simulink model "CONTROL_SYSTEM_V3"  (R2024a)
settings: Solver=FixedStepAuto  StartTime=0.0  StopTime=inf  FixedStep=0.01  RelTol=1e-3
values from neighbouring files (symbols this model uses):
  Beta1 = 3*Omega_o    (= 15)    [CONTROL_SYSTEM_VAR.m]
  Beta2 = 3*(Omega_o^2)    (= 75)    [CONTROL_SYSTEM_VAR.m]
  Beta3 = (Omega_o^3)    (= 125)    [CONTROL_SYSTEM_VAR.m]
  Desire_Max = 255    [CONTROL_SYSTEM_VAR.m]
  Desire_Min = 0    [CONTROL_SYSTEM_VAR.m]
  Direction_Pin = 1    [CONTROL_SYSTEM_VAR.m]
  EN_Pin = 0    [CONTROL_SYSTEM_VAR.m]
  J_aet = 0.0035    [CONTROL_SYSTEM_VAR.m]
  Kd = 2    [CONTROL_SYSTEM_VAR.m]
  Ki = 4    [CONTROL_SYSTEM_VAR.m]
  Kn = 0.1    [CONTROL_SYSTEM_VAR.m]
  Kp = 1.4    [CONTROL_SYSTEM_VAR.m]
  omga_c = 10    [CONTROL_SYSTEM_VAR.m]
  roa = 0.24    [CONTROL_SYSTEM_VAR.m]
undefined symbols (not defined in the file or in its folder): sigbuilder_block
libraries: arduinolib x30, simulink_extras x14, simulink x5, slpidlib x4, SignalEditorBlockLib x3, slctrl_adaptive x2, spsOnDelayLib x2, slctrl_autotuning x2
(part 1 of 5)
settings Model: ExtModeTrigDuration=2  Creator=Banana444  LastModifiedBy=Banana444
settings SolverCC: AutoInsertRateTranBlk=on
settings OptimizationCC: EnhancedBackFolding=on  PassReuseOutputArgsAs=Individual arguments  ZeroExternalMemoryAtStartup=off  ZeroInternalMemoryAtStartup=off  MaxStackSize=64  OptimizeBlockOrder=speed  DifferentSizesBufferReuse=on  OptimizationCustomize=off  EfficientTunableParamExpr=on
settings DebuggingCC: ParameterTunabilityLossMsg=error
settings HardwareCC: ProdBitPerPointer=32  ProdBitPerSizeT=32  ProdBitPerPtrDiffT=32  ProdLargestAtomicInteger=Long  ProdLargestAtomicFloat=Double  ProdWordSize=32  ProdHWDeviceType=ARM Compatible->ARM Cortex
settings SFSimCC: MATLABDynamicMemAlloc=off
settings RTWCC: Description=Embedded Coder  SystemTargetFile=ert.tlc  HardwareBoard=ESP32-WROOM(Arduino Compatible)  TLCOptions="-aInlineSetEventsForThisBaseRateFcn=TLC_FALSE -aSuppressMultiTaskScheduler=TLC_FALSE  -aRateBasedStepFcn=0"  TemplateMakefile=ert_default_tmf  Toolchain=ESP32
settings CodeAppCC: ForceParamTrailComments=on  IgnoreCustomStorageClasses=off  OperatorAnnotations=on  SimulinkDataObjDesc=on  SFDataObjDesc=on  InsertBlockDesc=on
settings ERTTargetCC: SupportContinuousTime=on  SupportVariableSizeSignals=on  ExtModeTransport=3  ExtModeStaticAlloc=on  ExtModeAutomaticAllocSize=off  ExtModeStaticAllocSize=65536  ExtModeMexFile=ext_xcp  ExtModeIntrfLevel=Level2 - Open

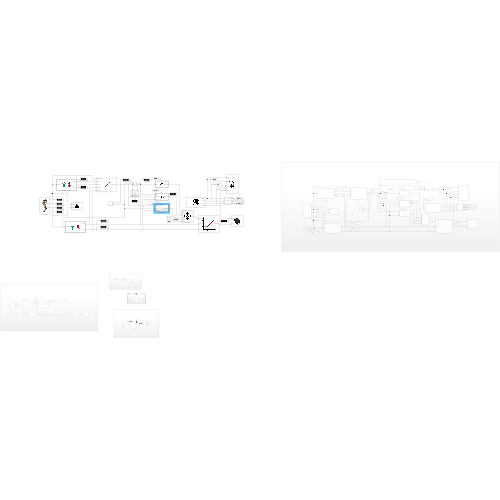
[thumbnail: Simulink's stored preview of the top-level diagram]
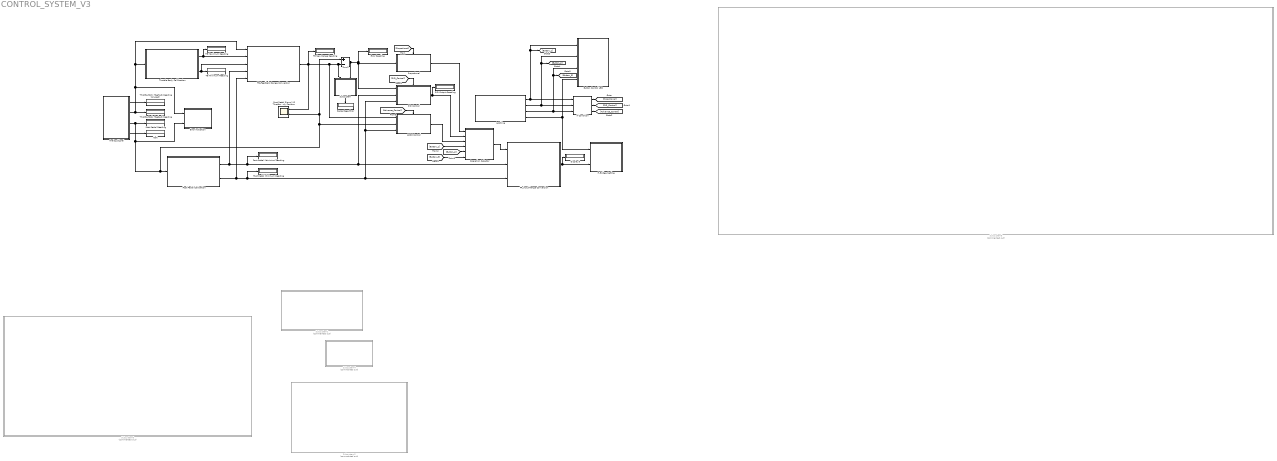
== system CONTROL_SYSTEM_V3 ==
  ADRC Control : Subsystem
  Analog Signal : Subsystem
      mask Display: image('Capture.JPG', [0,0,0,0,80,80]);
  Button Control LED : Subsystem
      mask Display: image('LED.png', [0,0,0,0,80,80]);
  Display3 : Display
      settings: Decimation=2
  Error Indication : Subsystem
      settings: PortSchema="{\"entries\":[{\"content\":{\"sides\":[{\"content\":{},\"type\":\"ConnectorPlacement.EquallySpacedRectSide\",\"uuid\":\"6bb27259-0fc4-412b-bd28-187413250838\"},{\"content\":{\"connectorIds\":[\"In1\",\"In2\"],\"side\":\"RIGHT\"},\"type\":\"ConnectorPlacement.EquallySpacedRectSide\",\"uuid\":\"b38a583a-7cdb-4b72-8a0e-445370b0f03f\"},{\"content\":{\"side\":\"TOP\"},\"type\":\"ConnectorPlacement.EquallySpacedRectSide\",\"uuid\":\"477ad40e-8e68-4653-afaf-50b4ab734c9d\"}]},\"type\":\"ConnectorPlacement.EquallySpacedConnector\",\"uuid\":\"474c0f68-6b48-44ee-b6ec-af4e49acdc40\"}],\"packageUris\":[\"http://schema.mathworks.com/mf0/Connector/R2020b\"],\"version\":\"1.0\"}"
      mask Display: image('Waring.png', [0,0,0,0,80,80]);
  Error Reading : Display
      settings: Decimation=2
  FP_Input Range Conversion : Subsystem
      mask Display: image('Interpolation.png', [0,0,0,0,80,80]);
  Foot Pedal Calibration : MATLAB Function  TreatAsAtomicUnit=on
  Foot Pedal Maximum Reading : Display
      settings: Decimation=2
  Foot Pedal Minimum Reading : Display
      settings: Decimation=2
  Foot Pedal Reading : Display
      settings: Decimation=2
  Foot Pedal Signal VS Throttle Body Position : Scope  NumInputPorts=2
  H-Bridge Setting : Subsystem
      mask Display: image('H-Bridge-removebg-preview.png', [0,0,0,0,80,80]);
  If Condition : If  NumInputs=3  IfExpression=u1 == 1  ElseIfExpressions=u2 == 1, u3 == 1  ShowElse=off
  Latching : Subsystem
      mask Display: image('Switch.png', [0,0,0,0,80,80]);
  NaN : Display
      settings: Decimation=2
  Operation Selector : Subsystem
      mask Display: image('Decision.png', [0,0,0,0,80,80]);
  PID Control : Subsystem
      mask Display: image('PID.PNG', [0,0,0,0,50,50]);
  PID Output Reading : Display
      settings: Decimation=2
  Percentage Error : Display
      settings: Decimation=2
  Propotional : Subsystem  TreatAsAtomicUnit=on
      mask Display: image('Propotional.png', [0,0,0,0,80,80]);
  Subsystem : Subsystem
      settings: PortSchema="{\"entries\":[{\"content\":{\"sides\":[{\"content\":{},\"type\":\"ConnectorPlacement.EquallySpacedRectSide\",\"uuid\":\"06ab9b8c-dc11-4e78-9aea-2a49b899d383\"},{\"content\":{\"side\":\"RIGHT\"},\"type\":\"ConnectorPlacement.EquallySpacedRectSide\",\"uuid\":\"ea81575a-6f3e-44ea-98d6-a15110b05ea2\"},{\"content\":{\"connectorIds\":[\"In1\",\"In2\"],\"side\":\"TOP\"},\"type\":\"ConnectorPlacement.EquallySpacedRectSide\",\"uuid\":\"b4582e74-93d2-4cba-bd7b-a3215d2fef1c\"},{\"content\":{\"connectorIds\":[\"Out1\"],\"side\":\"BOTTOM\"},\"type\":\"ConnectorPlacement.EquallySpacedRectSide\",\"uuid\":\"d3012ec7-4a68-4cee-bd0d-e63c4f089545\"}]},\"type\":\"ConnectorPlacement.EquallySpacedConnector\",\"uuid\":\"85ff3d74-6a46-44e9-8a38-f9999c5d3ee8\"}],\"packageUris\":[\"http://schema.mathworks.com/mf0/Connector/R2020b\"],\"version\":\"1.0\"}"
  Subsystem1 : Subsystem  Commented=on
  Subsystem2 : Subsystem  Commented=on
  Subsystem4 : Subsystem  Commented=on
  Subsystem5 : Subsystem  Commented=on
  Subsystem6 : Subsystem  Commented=on
  Sum2 : Sum  Inputs=+-
  TB Maximum Reading : Display
      settings: Decimation=2
  TB Minimum Reading : Display
      settings: Decimation=2
  TB New Range Reading : Display
      settings: Decimation=2
  TB_Feedbakc Range Conversion : Subsystem
      mask Display: image('Interpolation.png', [0,0,0,0,80,80]);
  Throttle Body Callibration : MATLAB Function  TreatAsAtomicUnit=on
  Throttle Body Feeback Reading : Display
      settings: Decimation=2
  Throttle Body Feeback Reading (Unused) : Display
      settings: Decimation=2
  wires:
  ADRC Control/1(ADRC Output) -> Operation Selector/3(Advanced Control)
  Propotional/1(Propotional) -> Operation Selector/1(Propotional)
  [Button_1] -> Operation Selector/4(Switch 1)
  Subsystem/1(Percentage Error) -> Percentage Error/1  "Percentage Error"
  Latching/3(Button 3) -> If Condition/3, [Button_3], Button Control LED/3(Button 3)
  [Advance_Control] -> ADRC Control/Action
  If Condition/2 -> [PID_Control]
  If Condition/1 -> [Propotional]
  [Propotional] -> Propotional/Action
  [Button_3] -> Operation Selector/6(Switch 3)
  TB_Feedbakc Range Conversion/1(TB New Range) -> Sum2/2, Subsystem/1(Throttle Body Feedback), ADRC Control/1(Feedback), Foot Pedal Signal VS Throttle Body Position/1, TB New Range Reading/1  "Throttle Body Feedback"
  Sum2/1 -> PID Control/1(Error), Propotional/1(Error), Error Reading/1, Subsystem/2(In1)  "Error"
  Throttle Body Callibration/1(TB_maxVal) -> TB Maximum Reading/1, TB_Feedbakc Range Conversion/2(TB_maxVal)
  Operation Selector/1(Control Output) -> FP_Input Range Conversion/1(Control Output)
  PID Control/1(PID Output) -> Operation Selector/2(PID Output), PID Output Reading/1
  Analog Signal/3(PedalRange) -> ADRC Control/2(Desire), Foot Pedal Signal VS Throttle Body Position/2, Sum2/1, Foot Pedal Calibration/1(PedalRange), Error Indication/1(PedalRange), Foot Pedal Reading/1  "Foot Pedal Signal"
  Foot Pedal Calibration/1(FP_maxVal) -> FP_Input Range Conversion/2(FP_maxVal), PID Control/2(FP_maxVal), Foot Pedal Maximum Reading/1, TB_Feedbakc Range Conversion/4(FP_maxVal)
  [Button_2] -> Operation Selector/5(Switch 2)
  If Condition/3 -> [Advance_Control]
  Analog Signal/4(Out4) -> NaN/1
  FP_Input Range Conversion/1(0 - 255 Output) -> H-Bridge Setting/2(0 - 255), Display3/1
  Latching/1(Button 1) -> [Button_1], Button Control LED/1(Button 1), If Condition/1
  Foot Pedal Calibration/2(FP_minVal) -> FP_Input Range Conversion/3(FP_minVal), ADRC Control/3(FP_minVal), PID Control/3(FP_minVal), Foot Pedal Minimum Reading/1, TB_Feedbakc Range Conversion/5(FP_minVal)
  Analog Signal/1(Out1) -> Throttle Body Feeback Reading (Unused)/1
  [PID_Control] -> PID Control/Action
  Latching/4(Button 4) -> H-Bridge Setting/1(Calibration Mode), Button Control LED/4(Button 4)
  Analog Signal/2(TBRange) -> Throttle Body Feeback Reading/1, Error Indication/2(TBRange), Throttle Body Callibration/1(TB_Range), TB_Feedbakc Range Conversion/1(Control Output)
  Throttle Body Callibration/2(TB_minVal) -> TB Minimum Reading/1, TB_Feedbakc Range Conversion/3(TB_minVal)
  Latching/2(Button 2) -> [Button_2], Button Control LED/2(Bottun 2), If Condition/2

== system CONTROL_SYSTEM_V3/ADRC Control ==
  Feedback : Inport
  Desire : Inport  Port=2
  FP_minVal : Inport  Port=3
  Action Port : ActionPort  ActionPortLabel=elseif( u3 == 1)
  Active Disturbance Rejection Control : slctrl_adaptive/Active Disturbance Rejection Control  time_domain=continuous-time  Ts=-1  model_type=second-order  b0=1000  wc=5  wo=5*8  x0=0  ulim_checkbox=off  umax=inf  umin=-inf  xhat_checkbox=off
      settings: LibrarySourceBlock=slctrlblks/Adaptive Control/Active Disturbance Rejection Control
  Constant : Constant  Value=2
  Divide : Product  Inputs=*/
  Saturation Dynamic : simulink/Discontinuities/Saturation Dynamic  OutMin=[]  OutMax=[]  OutDataTypeStr=Inherit: Same as second input  OutDataType=fixdt(1, 16)  OutScaling=2^-10  DoSatur=off
  Subsystem : Subsystem  Commented=on
  Sum1 : Sum  Inputs=++|
  ADRC Output : Outport
  wires:
  FP_minVal/1 -> Saturation Dynamic/3
  Subsystem/1(V(t)) -> ?
  Sum1/1 -> Saturation Dynamic/1
  Constant/1 -> Divide/2
  Active Disturbance Rejection Control/1 -> Saturation Dynamic/2
  Feedback/1 -> Active Disturbance Rejection Control/2
  Desire/1 -> Divide/1, Sum1/2, Active Disturbance Rejection Control/1
  Saturation Dynamic/1 -> ADRC Output/1
  Divide/1 -> Sum1/1

== system CONTROL_SYSTEM_V3/Analog Signal ==
  note: Analog Read Custom Block reaading;
      | - Throttle Body Feedback (V1)
      | - Foot Padel Signal (V2)
  MATLAB System : MATLABSystem  System=ADS1115_Vread  SetGain=int16( 16 )  SampleTime=-1
      mask Type: ADS1115_Vread
      mask Display:
      | color('white');plot([100,100,100,100]*1,[100,100,100,100]*1);plot([100,100,100,100]*0,[100,100,100,100]*0);color('blue');text(38, 92, 'IO Device Builder','horizontalAlignment', 'right');
      | color('black');text(52,50,' ADS1115_Vread','horizontalAlignment','center');
      | port_label('output',1,'V0');port_label('output',2,'V1');port_label('output',3,'V2');port_label('output',4,'V3');
  Out1 : Outport
  TBRange : Outport  Port=2
  PedalRange : Outport  Port=3
  Out4 : Outport  Port=4
  wires:
  MATLAB System/1 -> Out1/1
  MATLAB System/3 -> PedalRange/1
  MATLAB System/2 -> TBRange/1
  MATLAB System/4 -> Out4/1

== system CONTROL_SYSTEM_V3/Button Control LED ==
  Button 1 : Inport
  Bottun 2 : Inport  Port=2
  Button 3 : Inport  Port=3
  Button 4 : Inport  Port=4
  Constant : Constant  Value=0
  Digital Output : arduinolib/Digital Output  pinNumber=27  Direction=output  blockPlatform=arduino
  Digital Output1 : arduinolib/Digital Output  pinNumber=26  Direction=output  blockPlatform=arduino
  Digital Output2 : arduinolib/Digital Output  pinNumber=25  Direction=output  blockPlatform=arduino
  Digital Output3 : arduinolib/Digital Output  pinNumber=33  Direction=output  blockPlatform=arduino
  Pulse Generator : DiscretePulseGenerator  PulseType=Time based  Period=0.5  PulseWidth=50
  Switch : Switch  Criteria=u2 ~= 0  SaturateOnIntegerOverflow=off  InputSameDT=off
  wires:
  Button 1/1 -> Digital Output/1
  Bottun 2/1 -> Digital Output1/1
  Button 3/1 -> Digital Output2/1
  Pulse Generator/1 -> Switch/1
  Button 4/1 -> Switch/2
  Constant/1 -> Switch/3
  Switch/1 -> Digital Output3/1

== system CONTROL_SYSTEM_V3/Error Indication ==
  PedalRange : Inport
  TBRange : Inport  Port=2
  Constant : Constant
  Constant1 : Constant  Value=0
  Constant2 : Constant
  Constant3 : Constant  Value=0
  Constant4 : Constant  Value=0
  Digital Output4 : arduinolib/Digital Output  pinNumber=32  Direction=output  blockPlatform=arduino
  OR : Logic  Operator=NAND  IconShape=distinctive  AllPortsSameDT=off  OutDataTypeStr=boolean
  Pulse Generator : DiscretePulseGenerator  PulseType=Time based  Period=0.1  PulseWidth=50
  Switch : Switch  Criteria=u2 > Threshold  SaturateOnIntegerOverflow=off  InputSameDT=off
  Switch2 : Switch  Criteria=u2 > Threshold  SaturateOnIntegerOverflow=off  InputSameDT=off
  Switch3 : Switch  Criteria=u2 > Threshold  SaturateOnIntegerOverflow=off  InputSameDT=off
  wires:
  Switch3/1 -> Digital Output4/1
  Pulse Generator/1 -> Switch3/1
  Constant3/1 -> Switch2/3
  Switch/1 -> OR/1
  Switch2/1 -> OR/2
  Constant2/1 -> Switch2/1
  Constant/1 -> Switch/1
  Constant1/1 -> Switch/3
  OR/1 -> Switch3/2
  PedalRange/1 -> Switch2/2
  TBRange/1 -> Switch/2
  Constant4/1 -> Switch3/3

== system CONTROL_SYSTEM_V3/FP_Input Range Conversion ==
  note: Interpolation Equation to convert one range of value to another.
      | In this case, convert value range of foot padle to value range of 0-255 (which is how Arduino output port reads)
  Control Output : Inport
  FP_maxVal : Inport  Port=2
  FP_minVal : Inport  Port=3
  Add2 : Sum  Inputs=+-
  Add3 : Sum  Inputs=+-
  Desire Max Value : Constant  Value=Desire_Max
  Desire Min Value : Constant  Value=Desire_Min
  Display1 : Display
  Display3 : Display
  Divide1 : Product  Inputs=*/
  Product1 : Product
  Subtract : Sum  Inputs=+-
  Sum : Sum
  0 - 255 Output : Outport
  wires:
  Control Output/1 -> Subtract/1
  FP_maxVal/1 -> Add3/1
  Add3/1 -> Divide1/2, Display3/1
  FP_minVal/1 -> Subtract/2, Add3/2
  Desire Min Value/1 -> Add2/2, Sum/1
  Subtract/1 -> Product1/2
  Desire Max Value/1 -> Add2/1
  Add2/1 -> Display1/1, Divide1/1
  Divide1/1 -> Product1/1
  Product1/1 -> Sum/2
  Sum/1 -> 0 - 255 Output/1

== system CONTROL_SYSTEM_V3/H-Bridge Setting ==
  note: The setup is for calibration the throttle body after pressing the calibration button (Button_4). This will force the throttle body to open for 2 seconds before it close
  note: Setting for H-Bridge to control the throttle body
      | Enable Pin = 0
      | Direction Pin = 1
  Calibration Mode : Inport
  0 - 255 : Inport  Port=2
  Constant : Constant  Value=0
  Digital Output : arduinolib/Digital Output  pinNumber=0  Direction=output  blockPlatform=arduino
  Digital Output1 : arduinolib/Digital Output  pinNumber=16  Direction=output  blockPlatform=arduino
  Direction Pin : Constant  Value=Direction_Pin
  Display3 : Display
  Display4 : Display
  Enable Pin : Constant  Value=EN_Pin
  Gain : Gain  Gain=100
  On Delay : spsOnDelayLib/On Delay  DelayType=On delay  delay=1  ic=0  Ts=0
  PWM : arduinolib/PWM  pinNumber=4  frequencyType=Specify  desiredFrequency=19000  achievableFrequency=19000
  Switch1 : Switch  Criteria=u2 ~= 0  SaturateOnIntegerOverflow=off  InputSameDT=off
  Switch2 : Switch  Criteria=u2 ~= 0  SaturateOnIntegerOverflow=off  InputSameDT=off
  wires:
  Enable Pin/1 -> Display4/1, Digital Output/1
  Direction Pin/1 -> Display3/1, Digital Output1/1
  Gain/1 -> Switch1/1
  Calibration Mode/1 -> On Delay/1, Switch1/2, Gain/1
  0 - 255/1 -> Switch1/3
  Switch1/1 -> Switch2/3
  Switch2/1 -> PWM/1
  On Delay/1 -> Switch2/2
  Constant/1 -> Switch2/1

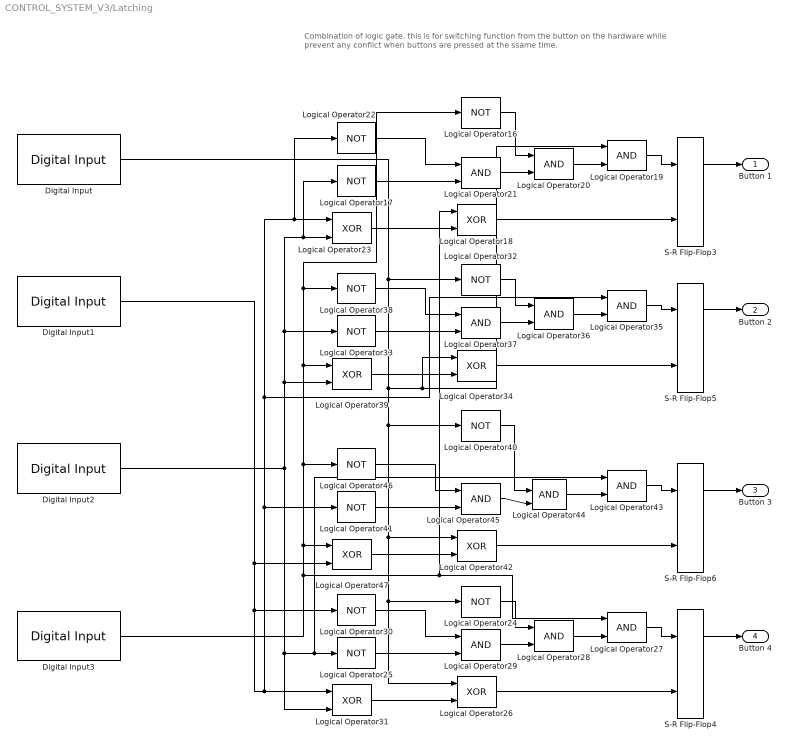
== system CONTROL_SYSTEM_V3/Latching ==
  note: Combination of logic gate. this is for switching function from the button on the hardware while prevent any conflict when buttons are pressed at the ssame time.
  Digital Input : arduinolib/Digital Input  pinNumber=36  mode=Default  Direction=input  SampleTime=-1  blockPlatform=arduino
  Digital Input1 : arduinolib/Digital Input  pinNumber=39  mode=Default  Direction=input  SampleTime=-1  blockPlatform=arduino
  Digital Input2 : arduinolib/Digital Input  pinNumber=34  mode=Default  Direction=input  SampleTime=-1  blockPlatform=arduino
  Digital Input3 : arduinolib/Digital Input  pinNumber=35  mode=Default  Direction=input  SampleTime=-1  blockPlatform=arduino
  Logical Operator{16..17,22,24..25,30,32..33,38,40..41,46} (12 alike) : Logic  Operator=NOT  IconShape=distinctive  AllPortsSameDT=off  OutDataTypeStr=boolean
  Logical Operator{18,23,26,31,34,39,42,47} (8 alike) : Logic  Operator=XOR  IconShape=distinctive  AllPortsSameDT=off  OutDataTypeStr=boolean
  Logical Operator{19..21,27..29,35..37,43..45} (12 alike) : Logic  IconShape=distinctive  AllPortsSameDT=off  OutDataTypeStr=boolean
  S-R Flip-Flop{3..6} (4 alike) : simulink_extras/Flip Flops/S-R Flip-Flop  initial_condition=0
  Button 1 : Outport
  Button 2 : Outport  Port=2
  Button 3 : Outport  Port=3
  Button 4 : Outport  Port=4
  wires:
  Digital Input2/1 -> Logical Operator25/1, Logical Operator43/1, Logical Operator31/2, Logical Operator17/1, Logical Operator23/2, Logical Operator33/1, Logical Operator39/2
  Digital Input3/1 -> Logical Operator16/1, Logical Operator38/1, Logical Operator39/1, Logical Operator46/1, Logical Operator47/1, Logical Operator18/1, Logical Operator27/1
  Digital Input1/1 -> Logical Operator47/2, Logical Operator30/1, Logical Operator41/1, Logical Operator22/1, Logical Operator23/1, Logical Operator35/1, Logical Operator31/1
  Logical Operator22/1 -> Logical Operator21/1
  Logical Operator17/1 -> Logical Operator21/2
  Logical Operator34/1 -> S-R Flip-Flop5/2
  Logical Operator33/1 -> Logical Operator37/2
  Logical Operator23/1 -> Logical Operator18/2
  Logical Operator39/1 -> Logical Operator34/2
  Logical Operator38/1 -> Logical Operator37/1
  Digital Input/1 -> Logical Operator40/1, Logical Operator24/1, Logical Operator26/1, Logical Operator42/1, Logical Operator19/1, Logical Operator34/1, Logical Operator32/1
  Logical Operator47/1 -> Logical Operator42/2
  Logical Operator46/1 -> Logical Operator45/1
  Logical Operator42/1 -> S-R Flip-Flop6/2
  Logical Operator41/1 -> Logical Operator45/2
  Logical Operator30/1 -> Logical Operator29/1
  Logical Operator26/1 -> S-R Flip-Flop4/2
  Logical Operator25/1 -> Logical Operator29/2
  Logical Operator36/1 -> Logical Operator35/2
  Logical Operator24/1 -> Logical Operator28/1
  Logical Operator31/1 -> Logical Operator26/2
  Logical Operator16/1 -> Logical Operator20/1
  Logical Operator35/1 -> S-R Flip-Flop5/1
  Logical Operator21/1 -> Logical Operator20/2
  Logical Operator19/1 -> S-R Flip-Flop3/1
  Logical Operator18/1 -> S-R Flip-Flop3/2
  Logical Operator29/1 -> Logical Operator28/2
  Logical Operator32/1 -> Logical Operator36/1
  Logical Operator37/1 -> Logical Operator36/2
  S-R Flip-Flop3/1 -> Button 1/1
  Logical Operator40/1 -> Logical Operator44/1
  Logical Operator45/1 -> Logical Operator44/2
  Logical Operator20/1 -> Logical Operator19/2
  Logical Operator43/1 -> S-R Flip-Flop6/1
  Logical Operator44/1 -> Logical Operator43/2
  Logical Operator27/1 -> S-R Flip-Flop4/1
  Logical Operator28/1 -> Logical Operator27/2
  S-R Flip-Flop5/1 -> Button 2/1
  S-R Flip-Flop6/1 -> Button 3/1
  S-R Flip-Flop4/1 -> Button 4/1

== system CONTROL_SYSTEM_V3/Operation Selector ==
  note: As the output of button is binary, therefore there are either 0 or 1. the simple equation for this is (Button_1 * 1) + (Button_2 * 2) + (Button_3 * 3) = Desired Mode
  note: Switch condition:
      | If the first button is pressed (output = 1), the system will run "No Control" mode
      | If the second button is pressed (output = 2), the system will run "PID Control" Mode
      | If the third button is pressed (output = 3), the system will run "Advanced Control" Mode
  Propotional : Inport
  PID Output : Inport  Port=2
  Advanced Control : Inport  Port=3
  Switch 1 : Inport  Port=4
  Switch 2 : Inport  Port=5
  Switch 3 : Inport  Port=6
  Add : Sum  Inputs=+++
  Multiply : Gain
  Multiply1 : Gain  Gain=2
  Multiply2 : Gain  Gain=3
  Multiport Switch : MultiPortSwitch  DiagnosticForDefault=None  SaturateOnIntegerOverflow=off  InputSameDT=off
  Control Output : Outport
  wires:
  Propotional/1 -> Multiport Switch/2
  Multiply/1 -> Add/1
  Multiply2/1 -> Add/3
  Add/1 -> Multiport Switch/1
  Switch 1/1 -> Multiply/1
  Multiply1/1 -> Add/2
  Switch 2/1 -> Multiply1/1
  Switch 3/1 -> Multiply2/1
  Advanced Control/1 -> Multiport Switch/4
  PID Output/1 -> Multiport Switch/3
  Multiport Switch/1 -> Control Output/1

== system CONTROL_SYSTEM_V3/PID Control ==
  note: PID control, with the saturation block to control the integral wind-up or any over shooting
      | the value of 0.01 is to give a room for slight over shooting value
  Error : Inport
  FP_maxVal : Inport  Port=2
  FP_minVal : Inport  Port=3
  Action Port : ActionPort  ActionPortLabel=elseif(u2 == 1)
  Constant : Constant  Value=0.01
  Derivative : Derivative  Commented=on
  Gain : Gain  Commented=on  Gain=5
  Gain1 : Gain  Commented=on  Gain=0.1
  PID Controller1 : slpidlib/PID Controller  Controller=PID  Form=Parallel  TimeDomain=Continuous-time  UseExternalTs=off  SampleTime=-1  IntegratorMethod=Forward Euler  FilterMethod=Forward Euler  ControllerParametersSource=internal  P=Kp  I=Ki  UseKiTs=off  D=Kd  UseExternalDerivativeSource=off  N=Kn  UseFilter=on  TunerSelectOption=Transfer Function Based (PID Tuner App)  InitialConditionSource=internal  InitialConditionForIntegrator=0  InitialConditionForFilter=0  DifferentiatorICPrevScaledInput=0  ExternalReset=none  TrackingMode=off  Kt=1  LimitOutput=off  SatLimitsSource=internal  UpperSaturationLimit=inf  LowerSaturationLimit=-inf  LinearizeAsGain=on  AntiWindupMode=none  Kb=1  LimitIntegrator=off  UpperIntegratorSaturationLimit=inf  LowerIntegratorSaturationLimit=-inf  POutMin=[]  POutMax=[]  IOutMin=[]  IOutMax=[]  DOutMin=[]  DOutMax=[]  NOutMin=[]  NOutMax=[]  SumOutMin=[]  SumOutMax=[]  SaturationOutMin=[]  SaturationOutMax=[]  PParamMin=[]  PParamMax=[]  IParamMin=[]  IParamMax=[]  DParamMin=[]  DParamMax=[]  NParamMin=[]  NParamMax=[]  KbParamMin=[]  KbParamMax=[]  KtParamMin=[]  KtParamMax=[]  KbOutMin=[]  KbOutMax=[]  KtOutMin=[]  KtOutMax=[]  IntegratorOutMin=[]  IntegratorOutMax=[]  FilterOutMin=[]  FilterOutMax=[]  SumI1OutMin=[]  SumI1OutMax=[]  SumI2OutMin=[]  SumI2OutMax=[]  SumI3OutMin=[]  SumI3OutMax=[]  SumI4OutMin=[]  SumI4OutMax=[]  SumDOutMin=[]  SumDOutMax=[]  DifferentiatorOutMin=[]  DifferentiatorOutMax=[]  FilterDiffOutCoefMin=[]  FilterDiffOutCoefMax=[]  ReciprocalOutMin=[]  ReciprocalOutMax=[]  SumDenOutMin=[]  SumDenOutMax=[]  SumNumOutMin=[]  SumNumOutMax=[]  DivideOutMin=[]  DivideOutMax=[]  UdiffTsProdOutMin=[]  UdiffTsProdOutMax=[]  NTsProdOutMin=[]  NTsProdOutMax=[]  UintegralTsProdOutMin=[]  UintegralTsProdOutMax=[]  UngainTsProdOutMin=[]  UngainTsProdOutMax=[]  ClampingZeroOutDataTypeStr=Inherit: Inherit via back propagation  ClampingZeroOutMin=[]  ClampingZeroOutMax=[]  FilterDenConstantOutDataTypeStr=Inherit: Inherit via back propagation  FilterDenConstantOutMin=[]  FilterDenConstantOutMax=[]  PCopyOutDataTypeStr=Inherit: Inherit via back propagation  PCopyOutMin=[]  PCopyOutMax=[]  NCopyOutDataTypeStr=Inherit: Inherit via back propagation  NCopyOutMin=[]  NCopyOutMax=[]  IntegratorContinuousStateAttributes=''  IntegratorStateMustResolveToSignalObject=off  IntegratorRTWStateStorageClass=Auto  FilterContinuousStateAttributes=''  FilterStateMustResolveToSignalObject=off  FilterRTWStateStorageClass=Auto  ParallelPVariant=InternalParameters  IdealPVariant=Disabled  IVariant=InternalParameters  DVariant=InternalParameters  IntegratorVariant=Continuous  SatVariant=Disabled  AWVariant=Passthrough  PCopyVariant=Disabled  TRVariant=Disabled  FdbkBlocksVariant=Forward  IdealPFdbkVariant=Disabled  SatFdbkVariant=Disabled  DerivativeFilterVariant=ContFilter  NVariant=InternalParameters  NCopyVariant=Disabled  FilterICVariant=InternalICsFilter  IntegratorICVariant=InternalICs  ExternalResetVariant=Disabled  TRSumVariant=Passthrough  SumFdbkVariant=Disabled  SumVariant=Sum_PID  TsampFilterVariant=InternalTs  TsampNgainVariant=Passthrough  TsampIntegralVariant=Disabled_SignalSpec  ExternalSaturationOutDataTypeStr=Inherit: Same as second input  DerivativeSourceVariant=ErrorSignal
  Saturation Dynamic : simulink/Discontinuities/Saturation Dynamic  OutMin=[]  OutMax=[]  OutDataTypeStr=Inherit: Same as second input  OutDataType=fixdt(1, 16)  OutScaling=2^-10  DoSatur=off
  Sign : Signum  Commented=on
  Sum : Sum  Commented=on  Inputs=|++
  Sum1 : Sum  Inputs=++|
  PID Output : Outport
  wires:
  Saturation Dynamic/1 -> PID Output/1
  FP_minVal/1 -> Saturation Dynamic/3
  Sum1/1 -> Saturation Dynamic/1
  Constant/1 -> Sum1/1
  FP_maxVal/1 -> Sum1/2
  PID Controller1/1 -> Saturation Dynamic/2
  Error/1 -> PID Controller1/1
  Sign/1 -> Gain1/1
  Sum/1 -> Sign/1
  Gain/1 -> Sum/1
  Derivative/1 -> Sum/2

== system CONTROL_SYSTEM_V3/Propotional ==
  Error : Inport
  Action Port : ActionPort  ActionPortLabel=if(u1 == 1)
  Propotional : Outport
  wires:
  Error/1 -> Propotional/1

== system CONTROL_SYSTEM_V3/Subsystem ==
  Throttle Body Feedback : Inport
  In1 : Inport  Port=2
  Abs : Abs  SaturateOnIntegerOverflow=off
  Divide : Product  Inputs=*/
  Gain : Gain  Gain=100
  Percentage Error : Outport
  wires:
  Divide/1 -> Abs/1
  Gain/1 -> Percentage Error/1  "Percentage Error"
  Abs/1 -> Gain/1
  In1/1 -> Divide/1
  Throttle Body Feedback/1 -> Divide/2

== system CONTROL_SYSTEM_V3/Subsystem1 ==
  In1 : Inport
  Pedal_Val : Inport  Port=2
  Constant : Constant  Value=0
  Constant1 : Constant
  Constant2 : Constant  Value=0.02
  Detect Increase1 : simulink/Logic and Bit Operations/Detect Increase  vinit=0.0  OutDataTypeStr=boolean
  Display13 : Display
      settings: Decimation=2
  MATLAB Function : MATLAB Function  TreatAsAtomicUnit=on
  Relational Operator : RelationalOperator  OutDataTypeStr=boolean  RndMeth=Simplest  InputSameDT=off
  Switch : Switch  Criteria=u2 ~= 0  Threshold=1  SaturateOnIntegerOverflow=off  InputSameDT=off
  Desire_Val : Outport
  wires:
  MATLAB Function/1(Desire_Val) -> Desire_Val/1
  In1/1 -> Relational Operator/2
  Switch/1 -> Display13/1, [try]
  Detect Increase1/1 -> Switch/2
  Constant/1 -> Switch/1
  Constant2/1 -> Relational Operator/1
  Constant1/1 -> Switch/3
  Relational Operator/1 -> Detect Increase1/1
  Pedal_Val/1 -> MATLAB Function/1(Pedal_Val)
